simulink model "SEAMOUR_Sim"  (R2023a)
settings: Solver=ode4  StartTime=0.0  StopTime=12  FixedStep=simulation_ts  MaxStep=0.001  MinStep=0.0001  RelTol=1e-3  EnableMultiTasking=on
values from neighbouring files (symbols this model uses):
  Area_y = [0.0031581,0.024875,0.025026,0.021123,0.021123,0.025026,0.024875,0.037486]    [init_file.m]
  Area_z = [0.0031588,0.028932,0.035488,0.030129,0.030129,0.035488,0.028932,0.039984]    [init_file.m]
  Cd_y = [0.5645,0.5232,0.4085,0.3589,0.3589,0.40849,0.5232,0.4642]    [init_file.m]
  Cd_z = [0.5645,0.52,0.5843,0.533,0.533,0.5843,0.52,0.5238]    [init_file.m]
  Coeff = [xudot, yvdot, zwdot]    [init_file.m]
  gravity = 9.81    [init_file.m]
  m = (4*pi*rho*a*b*b)/3    (= 16.3133743522)    [init_file.m]
  offset = 0.002    [init_file.m]
  percent_y = Area_y/t_y    [init_file.m]
  percent_z = Area_z/t_z    [init_file.m]
  xudot = k1*m    [init_file.m]
undefined symbols (not defined in the file or in its folder): center_body, headmain, headmotorshield, headmount, hindconnection, hindcover, kx_lower, kx_upper, kz_lower, kz_upper, lefthindflipper, lefthindmotor, leftmotor1, leftmotor2, leftmotor3, lf_lower, lf_upper, rf_lower, rf_upper, righthindflipper, righthindmotor, rightmotor1, rightmotor2, rightmotor3, tailmotorshield, tailmount, X, Y, Z
libraries: nesl_utility x208, sm_lib x149
(part 7 of 7)

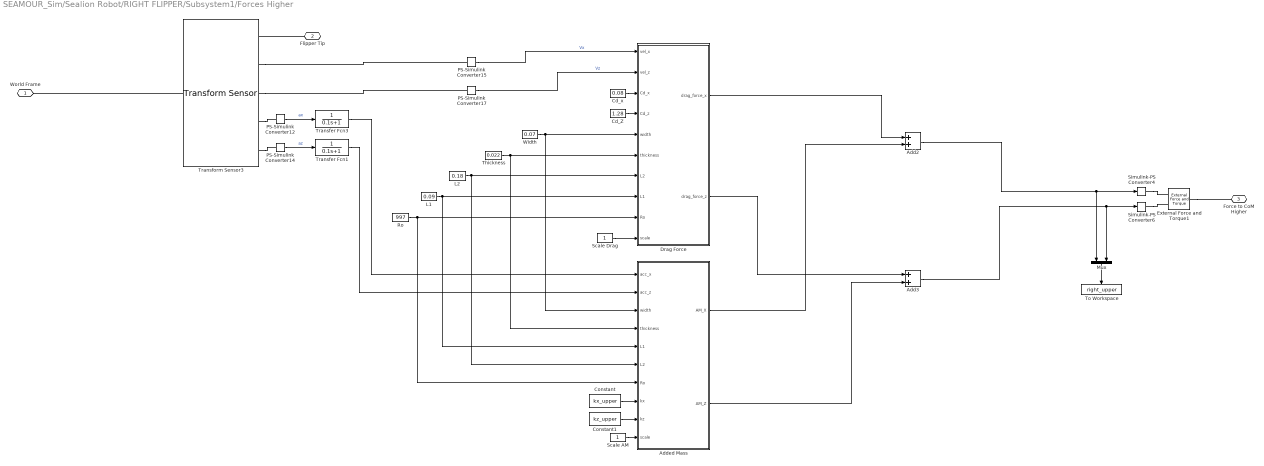
== system SEAMOUR_Sim/Sealion Robot/RIGHT FLIPPER/Subsystem1/Forces Higher ==
  Add2 : Sum
  Add3 : Sum
  Added Mass : MATLAB Function  TreatAsAtomicUnit=on
  Cd_Z : Constant  Value=1.28
  Cd_x : Constant  Value=0.08
  Constant : Constant  Value=kx_upper
  Constant1 : Constant  Value=kz_upper
  Drag Force : MATLAB Function  TreatAsAtomicUnit=on
  External Force and Torque1 : sm_lib/Forces and Torques/External Force and Torque  ForceResolutionFrame=AttachedFrame  EnableForceX=on  EnableForceY=off  EnableForceZ=on  EnableForce=off  TorqueResolutionFrame=AttachedFrame  EnableTorqueX=off  EnableTorqueY=off  EnableTorqueZ=off  EnableTorque=off
  L1 : Constant  Value=0.09
  L2 : Constant  Value=0.18
  Mux : Mux  Inputs=2
  PS-Simulink Converter{12,14..15,17} (4 alike) : nesl_utility/PS-Simulink Converter  PhysicalDomain=network_engine_domain  SubClassName=ps_output  LeftPortType=input  RightPortType=output  PseudoPeriodic=off  Frequencies=[]  VectorFormat=1-D array  Unit=1  AffineConversion=off
  Ro : Constant  Value=997
  Scale AM : Constant
  Scale Drag : Constant
  Simulink-PS Converter4 : nesl_utility/Simulink-PS Converter  PhysicalDomain=network_engine_domain  SubClassName=ps_input  LeftPortType=input  RightPortType=output  PseudoPeriodic=off  Frequencies=[]  NoiseDistribution=none  NoiseParameters=[]  Unit=1  AffineConversion=off  FilteringAndDerivatives=filter  SimscapeFilterOrder=2  InputFilterTimeConstant=0.001  UdotUserProvided=0
  Simulink-PS Converter6 : nesl_utility/Simulink-PS Converter  PhysicalDomain=network_engine_domain  SubClassName=ps_input  LeftPortType=input  RightPortType=output  PseudoPeriodic=off  Frequencies=[]  NoiseDistribution=none  NoiseParameters=[]  Unit=1  AffineConversion=off  FilteringAndDerivatives=filter  SimscapeFilterOrder=2  InputFilterTimeConstant=0.001  UdotUserProvided=0
  Thickness : Constant  Value=0.022
  To Workspace : ToWorkspace  VariableName=right_upper  SampleTime=-1
      settings: Save2DSignal=2-D array (concatenate along first dimension)
  Transfer Fcn1 : TransferFcn  Denominator=[0.1 1]
  Transfer Fcn3 : TransferFcn  Denominator=[0.1 1]
  Transform Sensor3 : sm_lib/Frames and Transforms/Transform Sensor  MeasurementFrame=NonRotatingFollower  RotationSequence=XYX  SenseAngle=off  SenseAxis=off  SenseQ=off  SenseR=off  SenseRotationSequence=off  SenseOmegaX=off  SenseOmegaY=off  SenseOmegaZ=off  SenseQDot=off  SenseRDot=off  SenseRotationSequenceDot=off  SenseAlphaX=off  SenseAlphaY=off  SenseAlphaZ=off  SenseQDDot=off  SenseRDDot=off  SenseX=off  SenseY=off  SenseZ=off  SenseRad=off  SenseAzim=off  SenseDist=off  SenseInc=off  SenseXDot=on  SenseYDot=off  SenseZDot=on  SenseRadDot=off  SenseAzimDot=off  SenseDistDot=off  SenseIncDot=off  SenseXDDot=on  SenseYDDot=off  SenseZDDot=on  SenseRadDDot=off  SenseAzimDDot=off  SenseDistDDot=off  SenseIncDDot=off
  Width : Constant  Value=0.07
  World Frame : PMIOPort  Side=Left
  Flipper Tip : PMIOPort  Port=2  Side=Right
  Force to CoM Higher : PMIOPort  Port=3  Side=Right
  wires:
  Constant1/1 -> Added Mass/9(kz)
  Added Mass/1(AM_X) -> Add2/2
  Mux/1 -> To Workspace/1
  Added Mass/2(AM_Z) -> Add3/2
  Scale AM/1 -> Added Mass/10(scale)
  PS-Simulink Converter14/1 -> Transfer Fcn1/1  "az"
  L2/1 -> Added Mass/6(L2), Drag Force/7(L2)
  Constant/1 -> Added Mass/8(kx)
  Cd_Z/1 -> Drag Force/4(Cd_z)
  Add2/1 -> Mux/1, Simulink-PS Converter4/1
  Drag Force/1(drag_force_x) -> Add2/1
  Transfer Fcn3/1 -> Added Mass/1(acc_x)
  Add3/1 -> Mux/2, Simulink-PS Converter6/1
  Width/1 -> Added Mass/3(width), Drag Force/5(width)
  Scale Drag/1 -> Drag Force/10(scale)
  Cd_x/1 -> Drag Force/3(Cd_x)
  Thickness/1 -> Added Mass/4(thickness), Drag Force/6(thickness)
  Transfer Fcn1/1 -> Added Mass/2(acc_z)
  PS-Simulink Converter17/1 -> Drag Force/2(vel_z)  "Vz"
  Ro/1 -> Added Mass/7(Ro), Drag Force/9(Ro)
  PS-Simulink Converter12/1 -> Transfer Fcn3/1  "ax"
  Drag Force/2(drag_force_z) -> Add3/1
  PS-Simulink Converter15/1 -> Drag Force/1(vel_x)  "Vx"
  L1/1 -> Added Mass/5(L1), Drag Force/8(L1)
  connections:
  Transform Sensor3/LConn1 -- World Frame/RConn1
  Flipper Tip/RConn1 -- Transform Sensor3/RConn1
  External Force and Torque1/RConn1 -- Force to CoM Higher/RConn1
  Transform Sensor3/RConn4 -- PS-Simulink Converter12/LConn1
  Transform Sensor3/RConn3 -- PS-Simulink Converter17/LConn1
  Simulink-PS Converter4/RConn1 -- External Force and Torque1/LConn1
  Transform Sensor3/RConn5 -- PS-Simulink Converter14/LConn1
  Simulink-PS Converter6/RConn1 -- External Force and Torque1/LConn2
  Transform Sensor3/RConn2 -- PS-Simulink Converter15/LConn1

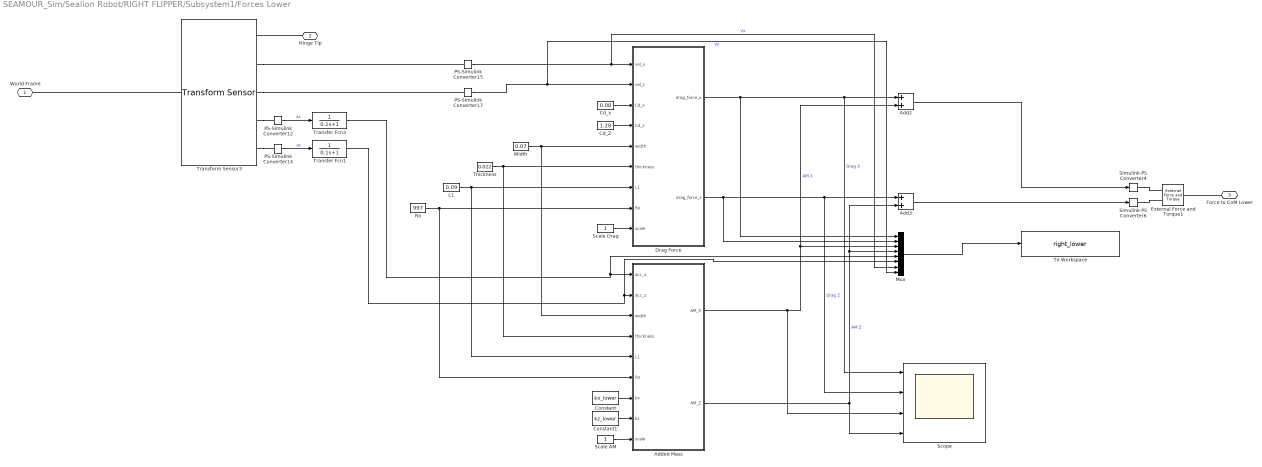
== system SEAMOUR_Sim/Sealion Robot/RIGHT FLIPPER/Subsystem1/Forces Lower ==
  Add2 : Sum
  Add3 : Sum
  Added Mass : MATLAB Function  TreatAsAtomicUnit=on
  Cd_Z : Constant  Value=1.28
  Cd_x : Constant  Value=0.08
  Constant : Constant  Value=kx_lower
  Constant1 : Constant  Value=kz_lower
  Drag Force : MATLAB Function  TreatAsAtomicUnit=on
  External Force and Torque1 : sm_lib/Forces and Torques/External Force and Torque  ForceResolutionFrame=AttachedFrame  EnableForceX=on  EnableForceY=off  EnableForceZ=on  EnableForce=off  TorqueResolutionFrame=AttachedFrame  EnableTorqueX=off  EnableTorqueY=off  EnableTorqueZ=off  EnableTorque=off
  L1 : Constant  Value=0.09
  Mux : Mux  Inputs=8
  PS-Simulink Converter{12,14..15,17} (4 alike) : nesl_utility/PS-Simulink Converter  PhysicalDomain=network_engine_domain  SubClassName=ps_output  LeftPortType=input  RightPortType=output  PseudoPeriodic=off  Frequencies=[]  VectorFormat=1-D array  Unit=1  AffineConversion=off
  Ro : Constant  Value=997
  Scale AM : Constant
  Scale Drag : Constant
  Scope : Scope  NumInputPorts=4
  Simulink-PS Converter4 : nesl_utility/Simulink-PS Converter  PhysicalDomain=network_engine_domain  SubClassName=ps_input  LeftPortType=input  RightPortType=output  PseudoPeriodic=off  Frequencies=[]  NoiseDistribution=none  NoiseParameters=[]  Unit=1  AffineConversion=off  FilteringAndDerivatives=filter  SimscapeFilterOrder=2  InputFilterTimeConstant=0.001  UdotUserProvided=0
  Simulink-PS Converter6 : nesl_utility/Simulink-PS Converter  PhysicalDomain=network_engine_domain  SubClassName=ps_input  LeftPortType=input  RightPortType=output  PseudoPeriodic=off  Frequencies=[]  NoiseDistribution=none  NoiseParameters=[]  Unit=1  AffineConversion=off  FilteringAndDerivatives=filter  SimscapeFilterOrder=2  InputFilterTimeConstant=0.001  UdotUserProvided=0
  Thickness : Constant  Value=0.022
  To Workspace : ToWorkspace  VariableName=right_lower  SampleTime=-1
      settings: Save2DSignal=2-D array (concatenate along first dimension)
  Transfer Fcn1 : TransferFcn  Denominator=[0.1 1]
  Transfer Fcn3 : TransferFcn  Denominator=[0.1 1]
  Transform Sensor3 : sm_lib/Frames and Transforms/Transform Sensor  MeasurementFrame=NonRotatingFollower  RotationSequence=XYX  SenseAngle=off  SenseAxis=off  SenseQ=off  SenseR=off  SenseRotationSequence=off  SenseOmegaX=off  SenseOmegaY=off  SenseOmegaZ=off  SenseQDot=off  SenseRDot=off  SenseRotationSequenceDot=off  SenseAlphaX=off  SenseAlphaY=off  SenseAlphaZ=off  SenseQDDot=off  SenseRDDot=off  SenseX=off  SenseY=off  SenseZ=off  SenseRad=off  SenseAzim=off  SenseDist=off  SenseInc=off  SenseXDot=on  SenseYDot=off  SenseZDot=on  SenseRadDot=off  SenseAzimDot=off  SenseDistDot=off  SenseIncDot=off  SenseXDDot=on  SenseYDDot=off  SenseZDDot=on  SenseRadDDot=off  SenseAzimDDot=off  SenseDistDDot=off  SenseIncDDot=off
  Width : Constant  Value=0.07
  World Frame : PMIOPort  Side=Left
  Hinge Tip : PMIOPort  Port=2  Side=Left
  Force to CoM Lower : PMIOPort  Port=3  Side=Right
  wires:
  Constant/1 -> Added Mass/7(kx)
  Drag Force/2(drag_force_z) -> Mux/2, Scope/2, Add3/1  "Drag Z"
  Transfer Fcn1/1 -> Mux/6, Added Mass/2(acc_z)
  Scale AM/1 -> Added Mass/9(scale)
  Transfer Fcn3/1 -> Mux/5, Added Mass/1(acc_x)
  Drag Force/1(drag_force_x) -> Mux/1, Scope/1, Add2/1  "Drag X"
  Add2/1 -> Simulink-PS Converter4/1
  PS-Simulink Converter14/1 -> Transfer Fcn1/1  "az"
  Added Mass/1(AM_X) -> Scope/3, Add2/2, Mux/3  "AM X"
  PS-Simulink Converter15/1 -> Mux/7, Drag Force/1(vel_x)  "Vx"
  Width/1 -> Added Mass/3(width), Drag Force/5(width)
  Mux/1 -> To Workspace/1
  Cd_Z/1 -> Drag Force/4(Cd_z)
  PS-Simulink Converter17/1 -> Mux/8, Drag Force/2(vel_z)  "Vz"
  Thickness/1 -> Added Mass/4(thickness), Drag Force/6(thickness)
  Ro/1 -> Added Mass/6(Ro), Drag Force/8(Ro)
  Add3/1 -> Simulink-PS Converter6/1
  Cd_x/1 -> Drag Force/3(Cd_x)
  L1/1 -> Drag Force/7(L1), Added Mass/5(L1)
  Scale Drag/1 -> Drag Force/9(scale)
  Added Mass/2(AM_Z) -> Add3/2, Mux/4, Scope/4  "AM Z"
  PS-Simulink Converter12/1 -> Transfer Fcn3/1  "ax"
  Constant1/1 -> Added Mass/8(kz)
  connections:
  Transform Sensor3/LConn1 -- World Frame/RConn1
  Hinge Tip/RConn1 -- Transform Sensor3/RConn1
  Transform Sensor3/RConn4 -- PS-Simulink Converter12/LConn1
  Force to CoM Lower/RConn1 -- External Force and Torque1/RConn1
  Transform Sensor3/RConn3 -- PS-Simulink Converter17/LConn1
  Transform Sensor3/RConn2 -- PS-Simulink Converter15/LConn1
  Simulink-PS Converter6/RConn1 -- External Force and Torque1/LConn2
  Transform Sensor3/RConn5 -- PS-Simulink Converter14/LConn1
  Simulink-PS Converter4/RConn1 -- External Force and Torque1/LConn1

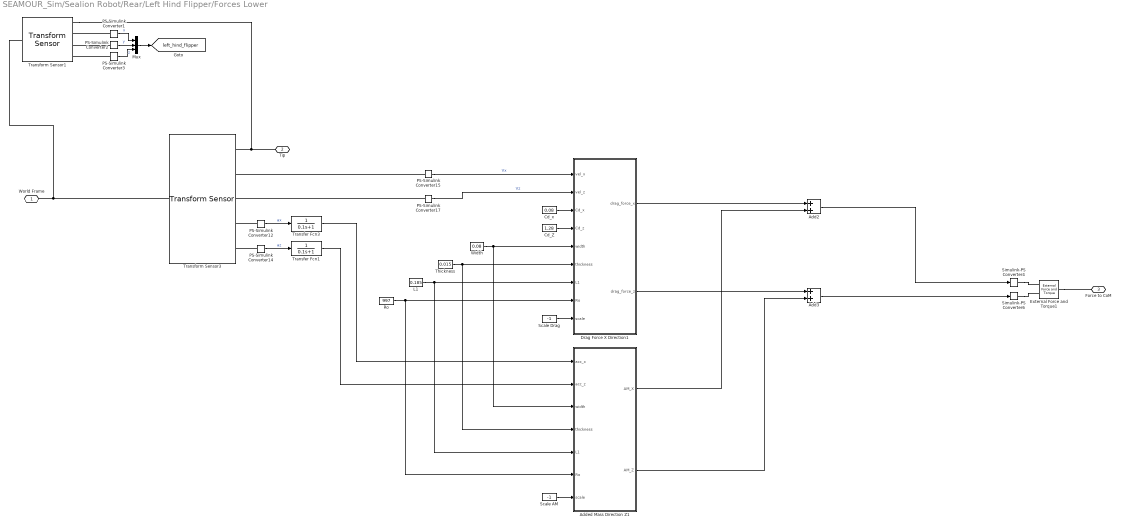
== system SEAMOUR_Sim/Sealion Robot/Rear/Left Hind Flipper/Forces Lower ==
  Add2 : Sum
  Add3 : Sum
  Added Mass Direction Z1 : MATLAB Function  TreatAsAtomicUnit=on
  Cd_Z : Constant  Value=1.28
  Cd_x : Constant  Value=0.08
  Drag Force X Direction1 : MATLAB Function  TreatAsAtomicUnit=on
  External Force and Torque1 : sm_lib/Forces and Torques/External Force and Torque  ForceResolutionFrame=AttachedFrame  EnableForceX=on  EnableForceY=off  EnableForceZ=on  EnableForce=off  TorqueResolutionFrame=AttachedFrame  EnableTorqueX=off  EnableTorqueY=off  EnableTorqueZ=off  EnableTorque=off
  L1 : Constant  Value=0.185
  Mux : Mux  Inputs=3
  PS-Simulink Converter{1..3,12,14..15,17} (7 alike) : nesl_utility/PS-Simulink Converter  PhysicalDomain=network_engine_domain  SubClassName=ps_output  LeftPortType=input  RightPortType=output  PseudoPeriodic=off  Frequencies=[]  VectorFormat=1-D array  Unit=1  AffineConversion=off
  Ro : Constant  Value=997
  Scale AM : Constant  Value=-1
  Scale Drag : Constant  Value=-1
  Simulink-PS Converter4 : nesl_utility/Simulink-PS Converter  PhysicalDomain=network_engine_domain  SubClassName=ps_input  LeftPortType=input  RightPortType=output  PseudoPeriodic=off  Frequencies=[]  NoiseDistribution=none  NoiseParameters=[]  Unit=1  AffineConversion=off  FilteringAndDerivatives=filter  SimscapeFilterOrder=2  InputFilterTimeConstant=0.001  UdotUserProvided=0
  Simulink-PS Converter6 : nesl_utility/Simulink-PS Converter  PhysicalDomain=network_engine_domain  SubClassName=ps_input  LeftPortType=input  RightPortType=output  PseudoPeriodic=off  Frequencies=[]  NoiseDistribution=none  NoiseParameters=[]  Unit=1  AffineConversion=off  FilteringAndDerivatives=filter  SimscapeFilterOrder=2  InputFilterTimeConstant=0.001  UdotUserProvided=0
  Thickness : Constant  Value=0.015
  Transfer Fcn1 : TransferFcn  Denominator=[0.1 1]
  Transfer Fcn3 : TransferFcn  Denominator=[0.1 1]
  Transform Sensor1 : sm_lib/Frames and Transforms/Transform Sensor  MeasurementFrame=NonRotatingFollower  RotationSequence=XYX  SenseAngle=off  SenseAxis=off  SenseQ=off  SenseR=off  SenseRotationSequence=off  SenseOmegaX=off  SenseOmegaY=off  SenseOmegaZ=off  SenseQDot=off  SenseRDot=off  SenseRotationSequenceDot=off  SenseAlphaX=off  SenseAlphaY=off  SenseAlphaZ=off  SenseQDDot=off  SenseRDDot=off  SenseX=on  SenseY=on  SenseZ=on  SenseRad=off  SenseAzim=off  SenseDist=off  SenseInc=off  SenseXDot=off  SenseYDot=off  SenseZDot=off  SenseRadDot=off  SenseAzimDot=off  SenseDistDot=off  SenseIncDot=off  SenseXDDot=off  SenseYDDot=off  SenseZDDot=off  SenseRadDDot=off  SenseAzimDDot=off  SenseDistDDot=off  SenseIncDDot=off
  Transform Sensor3 : sm_lib/Frames and Transforms/Transform Sensor  MeasurementFrame=NonRotatingFollower  RotationSequence=XYX  SenseAngle=off  SenseAxis=off  SenseQ=off  SenseR=off  SenseRotationSequence=off  SenseOmegaX=off  SenseOmegaY=off  SenseOmegaZ=off  SenseQDot=off  SenseRDot=off  SenseRotationSequenceDot=off  SenseAlphaX=off  SenseAlphaY=off  SenseAlphaZ=off  SenseQDDot=off  SenseRDDot=off  SenseX=off  SenseY=off  SenseZ=off  SenseRad=off  SenseAzim=off  SenseDist=off  SenseInc=off  SenseXDot=on  SenseYDot=off  SenseZDot=on  SenseRadDot=off  SenseAzimDot=off  SenseDistDot=off  SenseIncDot=off  SenseXDDot=on  SenseYDDot=off  SenseZDDot=on  SenseRadDDot=off  SenseAzimDDot=off  SenseDistDDot=off  SenseIncDDot=off
  Width : Constant  Value=0.08
  World Frame : PMIOPort  Side=Left
  Tip : PMIOPort  Port=2  Side=Right
  Force to CoM : PMIOPort  Port=3  Side=Right
  tag scope: left_hind_flipper=global
  wires:
  Thickness/1 -> Added Mass Direction Z1/4(thickness), Drag Force X Direction1/6(thickness)
  Scale AM/1 -> Added Mass Direction Z1/7(scale)
  Width/1 -> Added Mass Direction Z1/3(width), Drag Force X Direction1/5(width)
  L1/1 -> Drag Force X Direction1/7(L1), Added Mass Direction Z1/5(L1)
  PS-Simulink Converter17/1 -> Drag Force X Direction1/2(vel_z)  "Vz"
  Cd_Z/1 -> Drag Force X Direction1/4(Cd_z)
  PS-Simulink Converter14/1 -> Transfer Fcn1/1  "az"
  PS-Simulink Converter12/1 -> Transfer Fcn3/1  "ax"
  PS-Simulink Converter15/1 -> Drag Force X Direction1/1(vel_x)  "Vx"
  Cd_x/1 -> Drag Force X Direction1/3(Cd_x)
  Scale Drag/1 -> Drag Force X Direction1/9(scale)
  Drag Force X Direction1/1(drag_force_x) -> Add2/1
  Add3/1 -> Simulink-PS Converter6/1
  Add2/1 -> Simulink-PS Converter4/1
  Drag Force X Direction1/2(drag_force_z) -> Add3/1
  Transfer Fcn3/1 -> Added Mass Direction Z1/1(acc_x)
  Transfer Fcn1/1 -> Added Mass Direction Z1/2(acc_z)
  Ro/1 -> Added Mass Direction Z1/6(Ro), Drag Force X Direction1/8(Ro)
  Added Mass Direction Z1/1(AM_X) -> Add2/2
  Added Mass Direction Z1/2(AM_Z) -> Add3/2
  PS-Simulink Converter2/1 -> Mux/2  "y"
  PS-Simulink Converter3/1 -> Mux/3  "z"
  Mux/1 -> [left_hind_flipper]
  PS-Simulink Converter1/1 -> Mux/1  "x"
  connections:
  Transform Sensor3/LConn1 -- Transform Sensor1/LConn1 -- World Frame/RConn1
  External Force and Torque1/RConn1 -- Force to CoM/RConn1
  Simulink-PS Converter4/RConn1 -- External Force and Torque1/LConn1
  PS-Simulink Converter17/LConn1 -- Transform Sensor3/RConn3
  Simulink-PS Converter6/RConn1 -- External Force and Torque1/LConn2
  PS-Simulink Converter15/LConn1 -- Transform Sensor3/RConn2
  PS-Simulink Converter14/LConn1 -- Transform Sensor3/RConn5
  PS-Simulink Converter12/LConn1 -- Transform Sensor3/RConn4
  Tip/RConn1 -- Transform Sensor1/RConn1 -- Transform Sensor3/RConn1
  PS-Simulink Converter1/LConn1 -- Transform Sensor1/RConn2
  PS-Simulink Converter3/LConn1 -- Transform Sensor1/RConn4
  PS-Simulink Converter2/LConn1 -- Transform Sensor1/RConn3

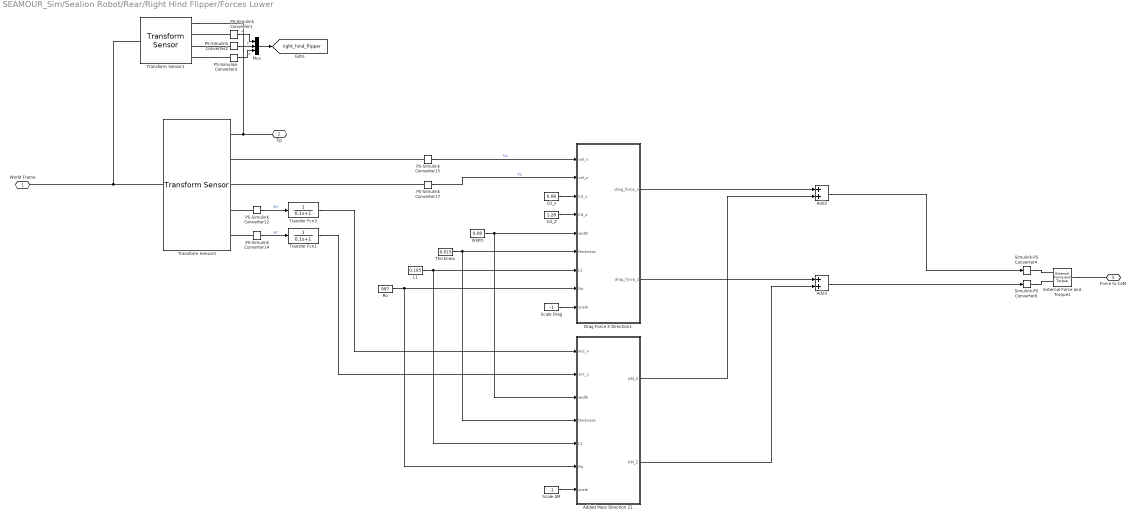
== system SEAMOUR_Sim/Sealion Robot/Rear/Right Hind Flipper/Forces Lower ==
  Add2 : Sum
  Add3 : Sum
  Added Mass Direction Z1 : MATLAB Function  TreatAsAtomicUnit=on
  Cd_Z : Constant  Value=1.28
  Cd_x : Constant  Value=0.08
  Drag Force X Direction1 : MATLAB Function  TreatAsAtomicUnit=on
  External Force and Torque1 : sm_lib/Forces and Torques/External Force and Torque  ForceResolutionFrame=AttachedFrame  EnableForceX=on  EnableForceY=off  EnableForceZ=on  EnableForce=off  TorqueResolutionFrame=AttachedFrame  EnableTorqueX=off  EnableTorqueY=off  EnableTorqueZ=off  EnableTorque=off
  L1 : Constant  Value=0.185
  Mux : Mux  Inputs=3
  PS-Simulink Converter{1..3,12,14..15,17} (7 alike) : nesl_utility/PS-Simulink Converter  PhysicalDomain=network_engine_domain  SubClassName=ps_output  LeftPortType=input  RightPortType=output  PseudoPeriodic=off  Frequencies=[]  VectorFormat=1-D array  Unit=1  AffineConversion=off
  Ro : Constant  Value=997
  Scale AM : Constant  Value=-1
  Scale Drag : Constant  Value=-1
  Simulink-PS Converter4 : nesl_utility/Simulink-PS Converter  PhysicalDomain=network_engine_domain  SubClassName=ps_input  LeftPortType=input  RightPortType=output  PseudoPeriodic=off  Frequencies=[]  NoiseDistribution=none  NoiseParameters=[]  Unit=1  AffineConversion=off  FilteringAndDerivatives=filter  SimscapeFilterOrder=2  InputFilterTimeConstant=0.001  UdotUserProvided=0
  Simulink-PS Converter6 : nesl_utility/Simulink-PS Converter  PhysicalDomain=network_engine_domain  SubClassName=ps_input  LeftPortType=input  RightPortType=output  PseudoPeriodic=off  Frequencies=[]  NoiseDistribution=none  NoiseParameters=[]  Unit=1  AffineConversion=off  FilteringAndDerivatives=filter  SimscapeFilterOrder=2  InputFilterTimeConstant=0.001  UdotUserProvided=0
  Thickness : Constant  Value=0.015
  Transfer Fcn1 : TransferFcn  Denominator=[0.1 1]
  Transfer Fcn3 : TransferFcn  Denominator=[0.1 1]
  Transform Sensor1 : sm_lib/Frames and Transforms/Transform Sensor  MeasurementFrame=NonRotatingFollower  RotationSequence=XYX  SenseAngle=off  SenseAxis=off  SenseQ=off  SenseR=off  SenseRotationSequence=off  SenseOmegaX=off  SenseOmegaY=off  SenseOmegaZ=off  SenseQDot=off  SenseRDot=off  SenseRotationSequenceDot=off  SenseAlphaX=off  SenseAlphaY=off  SenseAlphaZ=off  SenseQDDot=off  SenseRDDot=off  SenseX=on  SenseY=on  SenseZ=on  SenseRad=off  SenseAzim=off  SenseDist=off  SenseInc=off  SenseXDot=off  SenseYDot=off  SenseZDot=off  SenseRadDot=off  SenseAzimDot=off  SenseDistDot=off  SenseIncDot=off  SenseXDDot=off  SenseYDDot=off  SenseZDDot=off  SenseRadDDot=off  SenseAzimDDot=off  SenseDistDDot=off  SenseIncDDot=off
  Transform Sensor3 : sm_lib/Frames and Transforms/Transform Sensor  MeasurementFrame=NonRotatingFollower  RotationSequence=XYX  SenseAngle=off  SenseAxis=off  SenseQ=off  SenseR=off  SenseRotationSequence=off  SenseOmegaX=off  SenseOmegaY=off  SenseOmegaZ=off  SenseQDot=off  SenseRDot=off  SenseRotationSequenceDot=off  SenseAlphaX=off  SenseAlphaY=off  SenseAlphaZ=off  SenseQDDot=off  SenseRDDot=off  SenseX=off  SenseY=off  SenseZ=off  SenseRad=off  SenseAzim=off  SenseDist=off  SenseInc=off  SenseXDot=on  SenseYDot=off  SenseZDot=on  SenseRadDot=off  SenseAzimDot=off  SenseDistDot=off  SenseIncDot=off  SenseXDDot=on  SenseYDDot=off  SenseZDDot=on  SenseRadDDot=off  SenseAzimDDot=off  SenseDistDDot=off  SenseIncDDot=off
  Width : Constant  Value=0.08
  World Frame : PMIOPort  Side=Left
  Tip : PMIOPort  Port=2  Side=Right
  Force to CoM : PMIOPort  Port=3  Side=Right
  tag scope: right_hind_flipper=global
  wires:
  Thickness/1 -> Added Mass Direction Z1/4(thickness), Drag Force X Direction1/6(thickness)
  Scale AM/1 -> Added Mass Direction Z1/7(scale)
  Width/1 -> Added Mass Direction Z1/3(width), Drag Force X Direction1/5(width)
  L1/1 -> Drag Force X Direction1/7(L1), Added Mass Direction Z1/5(L1)
  PS-Simulink Converter17/1 -> Drag Force X Direction1/2(vel_z)  "Vz"
  Cd_Z/1 -> Drag Force X Direction1/4(Cd_z)
  PS-Simulink Converter14/1 -> Transfer Fcn1/1  "az"
  PS-Simulink Converter12/1 -> Transfer Fcn3/1  "ax"
  PS-Simulink Converter15/1 -> Drag Force X Direction1/1(vel_x)  "Vx"
  Cd_x/1 -> Drag Force X Direction1/3(Cd_x)
  Scale Drag/1 -> Drag Force X Direction1/9(scale)
  Drag Force X Direction1/1(drag_force_x) -> Add2/1
  Add3/1 -> Simulink-PS Converter6/1
  Add2/1 -> Simulink-PS Converter4/1
  Drag Force X Direction1/2(drag_force_z) -> Add3/1
  Transfer Fcn3/1 -> Added Mass Direction Z1/1(acc_x)
  Transfer Fcn1/1 -> Added Mass Direction Z1/2(acc_z)
  Ro/1 -> Added Mass Direction Z1/6(Ro), Drag Force X Direction1/8(Ro)
  Added Mass Direction Z1/1(AM_X) -> Add2/2
  Added Mass Direction Z1/2(AM_Z) -> Add3/2
  PS-Simulink Converter2/1 -> Mux/2  "y"
  PS-Simulink Converter1/1 -> Mux/1  "x"
  Mux/1 -> [right_hind_flipper]
  PS-Simulink Converter3/1 -> Mux/3  "z"
  connections:
  Transform Sensor3/LConn1 -- Transform Sensor1/LConn1 -- World Frame/RConn1
  External Force and Torque1/RConn1 -- Force to CoM/RConn1
  Simulink-PS Converter4/RConn1 -- External Force and Torque1/LConn1
  PS-Simulink Converter17/LConn1 -- Transform Sensor3/RConn3
  Simulink-PS Converter6/RConn1 -- External Force and Torque1/LConn2
  PS-Simulink Converter15/LConn1 -- Transform Sensor3/RConn2
  PS-Simulink Converter14/LConn1 -- Transform Sensor3/RConn5
  PS-Simulink Converter12/LConn1 -- Transform Sensor3/RConn4
  Tip/RConn1 -- Transform Sensor1/RConn1 -- Transform Sensor3/RConn1
  PS-Simulink Converter3/LConn1 -- Transform Sensor1/RConn4
  PS-Simulink Converter2/LConn1 -- Transform Sensor1/RConn3
  PS-Simulink Converter1/LConn1 -- Transform Sensor1/RConn2

== matlab function SEAMOUR_Sim/Sealion Robot/LEFT FLIPPER/Subsystem/Forces Lower/Added Mass Direction Z1 ==
  data: acc_x input; acc_z input; width input; thickness input; L1 input; Ro input; kx input; kz input; scale input; AM_X output; AM_Z output
function [AM_X, AM_Z]=Added_Mass_Lower(acc_x,acc_z,width,thickness,L1,Ro,kx,kz,scale)

X_Coeff=(1/4)*pi*Ro*kx*thickness^2*L1;
Z_Coeff=(1/4)*pi*Ro*kz*width^2*L1;

AM_X = -(1/2)*acc_x*L1*X_Coeff*scale;
AM_Z = -(1/2)*acc_z*L1*Z_Coeff*scale;

end

== matlab function SEAMOUR_Sim/Sealion Robot/LEFT FLIPPER/Subsystem/Forces Lower/Drag Force X Direction1 ==
  data: vel_x input; drag_force_x output; vel_z input; Cd_x input; Cd_z input; width input; thickness input; L1 input; Ro input; drag_force_z output; scale input
function [drag_force_x, drag_force_z]=...
    Drag_Force(vel_x,vel_z,Cd_x,Cd_z,width,thickness,L1,Ro,scale)

    drag_force_x=-(1/8)*Ro*Cd_x*thickness*vel_x*abs(vel_x)*(L1^2)*scale; 
    drag_force_z=-(1/8)*Ro*Cd_z*width*vel_z*abs(vel_z)*(L1^2)*scale; 
end

== matlab function SEAMOUR_Sim/Sealion Robot/RIGHT FLIPPER/Subsystem1/Forces Lower/Added Mass ==
  data: acc_x input; acc_z input; width input; thickness input; L1 input; Ro input; kx input; kz input; scale input; AM_X output; AM_Z output
function [AM_X, AM_Z]=Added_Mass_Lower(acc_x,acc_z,width,thickness,L1,Ro,kx,kz,scale)

X_Coeff=(1/4)*pi*Ro*kx*thickness^2*L1;
Z_Coeff=(1/4)*pi*Ro*kz*width^2*L1;

AM_X = -(1/2)*acc_x*L1*X_Coeff*scale;
AM_Z = -(1/2)*acc_z*L1*Z_Coeff*scale;

end

== matlab function SEAMOUR_Sim/Sealion Robot/RIGHT FLIPPER/Subsystem1/Forces Lower/Drag Force ==
  data: vel_x input; drag_force_x output; vel_z input; Cd_x input; Cd_z input; width input; thickness input; L1 input; Ro input; drag_force_z output; scale input
function [drag_force_x, drag_force_z]=...
    Drag_Force(vel_x,vel_z,Cd_x,Cd_z,width,thickness,L1,Ro,scale)

    drag_force_x=-(1/8)*Ro*Cd_x*thickness*vel_x*abs(vel_x)*(L1^2)*scale; 
    drag_force_z=-(1/8)*Ro*Cd_z*width*vel_z*abs(vel_z)*(L1^2)*scale; 
end

== matlab function SEAMOUR_Sim/Sealion Robot/Rear/Left Hind Flipper/Forces Lower/Added Mass Direction Z1 ==
  data: acc_x input; acc_z input; width input; thickness input; L1 input; Ro input; scale input; AM_X output; AM_Z output
function [AM_X, AM_Z]=Added_Mass(acc_x,acc_z,width,thickness,L1,Ro,scale)

AM_X = -4.75*Ro*(thickness/2)*acc_x*0.5*(L1^2)*scale;
AM_Z = -4.75*Ro*(width/2)*acc_z*0.5*(L1^2)*scale;

end

== matlab function SEAMOUR_Sim/Sealion Robot/Rear/Left Hind Flipper/Forces Lower/Drag Force X Direction1 ==
  data: vel_x input; drag_force_x output; vel_z input; Cd_x input; Cd_z input; width input; thickness input; L1 input; Ro input; drag_force_z output; scale input
function [drag_force_x, drag_force_z]=...
    Drag_Force(vel_x,vel_z,Cd_x,Cd_z,width,thickness,L1,Ro,scale)

    drag_force_x=-(1/8)*Ro*Cd_x*thickness*vel_x*abs(vel_x)*(L1^2)*scale; 
    drag_force_z=-(1/8)*Ro*Cd_z*width*vel_z*abs(vel_z)*(L1^2)*scale; 
end

== matlab function SEAMOUR_Sim/Sealion Robot/RIGHT FLIPPER/Subsystem1/Forces Higher/Added Mass ==
  data: acc_x input; acc_z input; width input; thickness input; L1 input; L2 input; Ro input; kx input; kz input; scale input; AM_X output; AM_Z output
function [AM_X, AM_Z]=Added_Mass_Lower(acc_x,acc_z,width,thickness,L1,L2,Ro,kx,kz,scale)

X_Coeff=(1/4)*pi*Ro*kx*thickness^2*L2;
Z_Coeff=(1/4)*pi*Ro*kz*width^2*L2;

AM_X = -((.5*L2^2+L1)*acc_x*X_Coeff)/(L2+L1)*scale;
AM_Z = -((.5*L2^2+L1)*acc_z*Z_Coeff)/(L2+L1)*scale;

end

== matlab function SEAMOUR_Sim/Sealion Robot/HEAD/Head/Subsystem/Added Mass F ==
  data: acc_y input; acc_z input; AM_Y output; Coeff input; percent_y input; AM_Z output; percent_z input
function [AM_Y,AM_Z]=Added_Mass(acc_y,acc_z,Coeff,percent_y,percent_z)

    AM_Y=-acc_y*Coeff(2)*percent_y(1);
    AM_Z=-acc_z*Coeff(3)*percent_z(1);

end

== matlab function SEAMOUR_Sim/Sealion Robot/Rear/Right Hind Flipper/Forces Lower/Added Mass Direction Z1 ==
  data: acc_x input; acc_z input; width input; thickness input; L1 input; Ro input; scale input; AM_X output; AM_Z output
function [AM_X, AM_Z]=Added_Mass(acc_x,acc_z,width,thickness,L1,Ro,scale)

AM_X = -4.75*Ro*(thickness/2)*acc_x*0.5*(L1^2)*scale;
AM_Z = -4.75*Ro*(width/2)*acc_z*0.5*(L1^2)*scale;

end

== matlab function SEAMOUR_Sim/Sealion Robot/Rear/Right Hind Flipper/Forces Lower/Drag Force X Direction1 ==
  data: vel_x input; drag_force_x output; vel_z input; Cd_x input; Cd_z input; width input; thickness input; L1 input; Ro input; drag_force_z output; scale input
function [drag_force_x, drag_force_z]=...
    Drag_Force(vel_x,vel_z,Cd_x,Cd_z,width,thickness,L1,Ro,scale)

    drag_force_x=-(1/8)*Ro*Cd_x*thickness*vel_x*abs(vel_x)*(L1^2)*scale; 
    drag_force_z=-(1/8)*Ro*Cd_z*width*vel_z*abs(vel_z)*(L1^2)*scale; 
end

== matlab function SEAMOUR_Sim/Sealion Robot/6 DoF Joint/MATLAB Function ==
  data: u input; y output
function y = toEuler(u)

y = quat2eul(u');
end

== matlab function SEAMOUR_Sim/Sealion Robot/HEAD/Head/Subsystem/Drag F ==
  data: vel_y input; vel_z input; D_Y output; Cd_y input; Cd_z input; Area_y input; Area_z input; D_Z output; scale input
function [D_Y,D_Z]=Drag_Force(vel_y,vel_z,Cd_y,Cd_z,Area_y,Area_z,scale)
ro=998;
D_Y = -.5*ro*Cd_y(1)*Area_y(1)*(abs(vel_y)*vel_y)*scale;
D_Z = -.5*ro*Cd_z(1)*Area_z(1)*(abs(vel_z)*vel_z)*scale;

end

== matlab function SEAMOUR_Sim/Sealion Robot/Rear/Tail Section Forces/Added Mass F ==
  data: acc_y input; acc_z input; AM_Y output; Coeff input; percent_y input; AM_Z output; percent_z input
function [AM_Y,AM_Z]=Added_Mass(acc_y,acc_z,Coeff,percent_y,percent_z)

    AM_Y=-acc_y*Coeff(2)*percent_y(8);
    AM_Z=-acc_z*Coeff(3)*percent_z(8);

end

== matlab function SEAMOUR_Sim/Sealion Robot/Distributed Forces/Distbuted Load In y and z directions/Subsystem/Drag F ==
  data: vel_y input; vel_z input; D_Y output; Cd_y input; Cd_z input; Area_y input; Area_z input; D_Z output
function [D_Y,D_Z]=Drag_Force(vel_y,vel_z,Cd_y,Cd_z,Area_y,Area_z)
ro=998;
D_Y = -.5*ro*Cd_y(2)*Area_y(2)*(abs(vel_y)*vel_y);
D_Z = -.5*ro*Cd_z(2)*Area_z(2)*(abs(vel_z)*vel_z);

end

== matlab function SEAMOUR_Sim/Sealion Robot/Distributed Forces/Distbuted Load In y and z directions/Subsystem1/Added Mass F ==
  data: acc_y input; acc_z input; AM_Y output; Coeff input; percent_y input; AM_Z output; percent_z input
function [AM_Y,AM_Z]=Added_Mass(acc_y,acc_z,Coeff,percent_y,percent_z)

    AM_Y=-acc_y*Coeff(2)*percent_y(3);
    AM_Z=-acc_z*Coeff(3)*percent_z(3);

end

== matlab function SEAMOUR_Sim/Sealion Robot/Rear/Tail Section Forces/Drag F ==
  data: vel_y input; vel_z input; D_Y output; Cd_y input; Cd_z input; Area_y input; Area_z input; D_Z output; scale input
function [D_Y,D_Z]=Drag_Force(vel_y,vel_z,Cd_y,Cd_z,Area_y,Area_z,scale)
ro=998;
D_Y = -.5*ro*Cd_y(8)*Area_y(8)*(abs(vel_y)*vel_y)*scale;
D_Z = -.5*ro*Cd_z(8)*Area_z(8)*(abs(vel_z)*vel_z)*scale;

end

== matlab function SEAMOUR_Sim/Sealion Robot/Distributed Forces/Distbuted Load In y and z directions/Subsystem1/Drag F ==
  data: vel_y input; vel_z input; D_Y output; Cd_y input; Cd_z input; Area_y input; Area_z input; D_Z output
function [D_Y,D_Z]=Drag_Force(vel_y,vel_z,Cd_y,Cd_z,Area_y,Area_z)
ro=998;
D_Y = -.5*ro*Cd_y(3)*Area_y(3)*(abs(vel_y)*vel_y);
D_Z = -.5*ro*Cd_z(3)*Area_z(3)*(abs(vel_z)*vel_z);

end

== matlab function SEAMOUR_Sim/Sealion Robot/Distributed Forces/Distbuted Load In y and z directions/Subsystem2/Added Mass F ==
  data: acc_y input; acc_z input; AM_Y output; Coeff input; percent_y input; AM_Z output; percent_z input
function [AM_Y,AM_Z]=Added_Mass(acc_y,acc_z,Coeff,percent_y,percent_z)

    AM_Y=-acc_y*Coeff(2)*percent_y(4);
    AM_Z=-acc_z*Coeff(3)*percent_z(4);

end

== matlab function SEAMOUR_Sim/Sealion Robot/Distributed Forces/Distbuted Load In y and z directions/Subsystem2/Drag F ==
  data: vel_y input; vel_z input; D_Y output; Cd_y input; Cd_z input; Area_y input; Area_z input; D_Z output
function [D_Y,D_Z]=Drag_Force(vel_y,vel_z,Cd_y,Cd_z,Area_y,Area_z)
ro=998;
D_Y = -.5*ro*Cd_y(4)*Area_y(4)*(abs(vel_y)*vel_y);
D_Z = -.5*ro*Cd_z(4)*Area_z(4)*(abs(vel_z)*vel_z);

end

== matlab function SEAMOUR_Sim/Sealion Robot/Distributed Forces/Distbuted Load In y and z directions/Subsystem3/Added Mass F ==
  data: acc_y input; acc_z input; AM_Y output; Coeff input; percent_y input; AM_Z output; percent_z input
function [AM_Y,AM_Z]=Added_Mass(acc_y,acc_z,Coeff,percent_y,percent_z)

    AM_Y=-acc_y*Coeff(2)*percent_y(5);
    AM_Z=-acc_z*Coeff(3)*percent_z(5);

end

== matlab function SEAMOUR_Sim/Sealion Robot/Distributed Forces/Distbuted Load In y and z directions/Subsystem3/Drag F ==
  data: vel_y input; vel_z input; D_Y output; Cd_y input; Cd_z input; Area_y input; Area_z input; D_Z output
function [D_Y,D_Z]=Drag_Force(vel_y,vel_z,Cd_y,Cd_z,Area_y,Area_z)
ro=998;
D_Y = -.5*ro*Cd_y(5)*Area_y(5)*(abs(vel_y)*vel_y);
D_Z = -.5*ro*Cd_z(5)*Area_z(5)*(abs(vel_z)*vel_z);

end

== matlab function SEAMOUR_Sim/Sealion Robot/RIGHT FLIPPER/Subsystem1/Forces Higher/Drag Force ==
  data: vel_x input; drag_force_x output; vel_z input; Cd_x input; Cd_z input; width input; thickness input; L2 input; L1 input; Ro input; drag_force_z output; scale input
function [drag_force_x, drag_force_z]=...
    Drag_Force(vel_x,vel_z,Cd_x,Cd_z,width,thickness,L2,L1,Ro,scale)

    drag_force_x=-0.5*Cd_x*Ro*thickness*(abs(vel_x)*(vel_x))/4*((L1+L2)^4-L1^4)/(L1+L2)^2*scale; 
    drag_force_z=-0.5*Cd_z*Ro*width*(abs(vel_z)*(vel_z))/4*((L1+L2)^4-L1^4)/(L1+L2)^2*scale; 

end

== matlab function SEAMOUR_Sim/Sealion Robot/Distributed Forces/Distbuted Load In y and z directions/Subsystem4/Added Mass F ==
  data: acc_y input; acc_z input; AM_Y output; Coeff input; percent_y input; AM_Z output; percent_z input
function [AM_Y,AM_Z]=Added_Mass(acc_y,acc_z,Coeff,percent_y,percent_z)

    AM_Y=-acc_y*Coeff(2)*percent_y(6);
    AM_Z=-acc_z*Coeff(3)*percent_z(6);

end

== matlab function SEAMOUR_Sim/Sealion Robot/Distributed Forces/Distbuted Load In y and z directions/Subsystem4/Drag F ==
  data: vel_y input; vel_z input; D_Y output; Cd_y input; Cd_z input; Area_y input; Area_z input; D_Z output
function [D_Y,D_Z]=Drag_Force(vel_y,vel_z,Cd_y,Cd_z,Area_y,Area_z)
ro=998;
D_Y = -.5*ro*Cd_y(6)*Area_y(6)*(abs(vel_y)*vel_y);
D_Z = -.5*ro*Cd_z(6)*Area_z(6)*(abs(vel_z)*vel_z);

end

== matlab function SEAMOUR_Sim/Sealion Robot/Distributed Forces/Distbuted Load In y and z directions/Subsystem5/Added Mass F ==
  data: acc_y input; acc_z input; AM_Y output; Coeff input; percent_y input; AM_Z output; percent_z input
function [AM_Y,AM_Z]=Added_Mass(acc_y,acc_z,Coeff,percent_y,percent_z)

    AM_Y=-acc_y*Coeff(2)*percent_y(7);
    AM_Z=-acc_z*Coeff(3)*percent_z(7);

end

== matlab function SEAMOUR_Sim/Sealion Robot/Distributed Forces/Distbuted Load In y and z directions/Subsystem5/Drag F ==
  data: vel_y input; vel_z input; D_Y output; Cd_y input; Cd_z input; Area_y input; Area_z input; D_Z output
function [D_Y,D_Z]=Drag_Force(vel_y,vel_z,Cd_y,Cd_z,Area_y,Area_z)
ro=998;
D_Y = -.5*ro*Cd_y(7)*Area_y(7)*(abs(vel_y)*vel_y);
D_Z = -.5*ro*Cd_z(7)*Area_z(7)*(abs(vel_z)*vel_z);

end

== matlab function SEAMOUR_Sim/Sealion Robot/Distributed Forces/Drag force in x direction/Drag Main ==
  data: vel input; Cd input; Area input; scale input; drag_force output
function drag_force=Drag_Force(vel,Cd,Area,scale)

    drag_force=-(1/2)*997*Cd*(Area)*...
        (abs(vel)*vel)*scale;

end

== matlab function SEAMOUR_Sim/Sealion Robot/Distributed Forces/Added Mass in X/Added Mass D ==
  data: acc_x input; Coeffx input; AM_x output; scale input
function AM_x =Added_Mass(acc_x,Coeffx,scale)

    AM_x=acc_x*Coeffx*scale;
end

== matlab function SEAMOUR_Sim/Sealion Robot/Distributed Forces/Distbuted Load In y and z directions/Subsystem/Added Mass F ==
  data: acc_y input; acc_z input; AM_Y output; Coeff input; percent_y input; AM_Z output; percent_z input
function [AM_Y,AM_Z]=Added_Mass(acc_y,acc_z,Coeff,percent_y,percent_z)

    AM_Y=-acc_y*Coeff(2)*percent_y(2);
    AM_Z=-acc_z*Coeff(3)*percent_z(2);

end

== matlab function SEAMOUR_Sim/Sealion Robot/LEFT FLIPPER/Subsystem/Forces Higher/Added Mass ==
  data: acc_x input; acc_z input; width input; thickness input; L1 input; L2 input; Ro input; kx input; kz input; scale input; AM_X output; AM_Z output
function [AM_X, AM_Z]=Added_Mass_Lower(acc_x,acc_z,width,thickness,L1,L2,Ro,kx,kz,scale)

X_Coeff=(1/4)*pi*Ro*kx*thickness^2*L2;
Z_Coeff=(1/4)*pi*Ro*kz*width^2*L2;

AM_X = -((.5*L2^2+L1)*acc_x*X_Coeff)/(L2+L1)*scale;
AM_Z = -((.5*L2^2+L1)*acc_z*Z_Coeff)/(L2+L1)*scale;

end

== matlab function SEAMOUR_Sim/Sealion Robot/LEFT FLIPPER/Subsystem/Forces Higher/Drag Force ==
  data: vel_x input; drag_force_x output; vel_z input; Cd_x input; Cd_z input; width input; thickness input; L2 input; L1 input; Ro input; drag_force_z output; scale input
function [drag_force_x, drag_force_z]=...
    Drag_Force(vel_x,vel_z,Cd_x,Cd_z,width,thickness,L2,L1,Ro,scale)

    drag_force_x=-0.5*Cd_x*Ro*thickness*(abs(vel_x)*(vel_x))/4*((L1+L2)^4-L1^4)/(L1+L2)^2*scale; 
    drag_force_z=-0.5*Cd_z*Ro*width*(abs(vel_z)*(vel_z))/4*((L1+L2)^4-L1^4)/(L1+L2)^2*scale; 

end
